simulink model "VSD_Model"  (R2022a)
settings: Solver=VariableStepAuto  StartTime=0.0  StopTime=60
values from neighbouring files (symbols this model uses):
  Bm = 7.33*10^-8/(2*pi)    (= 1.16660573286e-08)    [VSD_Motors_initialization.m]
  fit_Cp_tail = @(u)feval(f_Cp_tail,u)    [VSD_Propellerfitting_tail.m]
  fit_Ct_tail = @(u)feval(f_Ct_tail,u)    [VSD_Propellerfitting_tail.m]
  fit_Pe_tail = @(u)feval(f_Pe_tail,u)    [VSD_Propellerfitting_tail.m]
  fit_Tl_tail = @(u)feval(f_Tl_tail,u)    [VSD_Propellerfitting_tail.m]
  Jm = 1.72 *10^-6    (= 1.72e-06)    [VSD_Motors_initialization.m]
  Ke = Km    (= 0.00118)    [VSD_Motors_initialization.m]
  Km = 1.18*10^-3    (= 0.00118)    [VSD_Motors_initialization.m]
  La = 0.274*10^-3    (= 0.000274)    [VSD_Motors_initialization.m]
  Q = 1e-6    (= 1e-06)    [VSD_initialization.m]
  R = 0.486    [VSD_Motors_initialization.m]    (also in VSD_initialization.m = 0.001)
  Ts = 1e-4    (= 0.0001)    [VSD_initialization.m]    (also in myStateTransitionFcn.m = 0.01)
  x0 = [0;0;0;0;0;0;0;0;0;0;0;0]    [VSD_SystemCheck.m]    (also in VSD_initialization.m = [0,0,0,0,0,0,0,0,0,0,0,0])
undefined symbols (not defined in the file or in its folder): Continuous, Time
libraries: slpidlib x7, simulink x7, sharedTrackingLibrary x3, ctrlSharedLib x1
(part 2 of 2)

== system VSD_Model/Control Allocation Subsystem/DC Motors/Motor21 ==
  w1_ref : Inport
  Tload : Inport  Port=2
  DC Motor : Subsystem
  PID Controller : slpidlib/PID Controller  Controller=PID  Form=Parallel  TimeDomain=Continuous-time  UseExternalTs=off  SampleTime=-1  IntegratorMethod=Forward Euler  FilterMethod=Forward Euler  ControllerParametersSource=internal  P=0.0221631801492144  I=0.197988325342969  UseKiTs=off  D=-5.9672220338915e-06  N=3714.15375920925  UseFilter=on  TunerSelectOption=Transfer Function Based (PID Tuner App)  InitialConditionSource=internal  InitialConditionForIntegrator=0  InitialConditionForFilter=0  DifferentiatorICPrevScaledInput=0  ExternalReset=none  TrackingMode=off  Kt=1  LimitOutput=off  SatLimitsSource=internal  UpperSaturationLimit=inf  LowerSaturationLimit=-inf  LinearizeAsGain=on  AntiWindupMode=none  Kb=1  POutMin=[]  POutMax=[]  IOutMin=[]  IOutMax=[]  DOutMin=[]  DOutMax=[]  NOutMin=[]  NOutMax=[]  SumOutMin=[]  SumOutMax=[]  SaturationOutMin=[]  SaturationOutMax=[]  PParamMin=[]  PParamMax=[]  IParamMin=[]  IParamMax=[]  DParamMin=[]  DParamMax=[]  NParamMin=[]  NParamMax=[]  KbParamMin=[]  KbParamMax=[]  KtParamMin=[]  KtParamMax=[]  KbOutMin=[]  KbOutMax=[]  KtOutMin=[]  KtOutMax=[]  IntegratorOutMin=[]  IntegratorOutMax=[]  FilterOutMin=[]  FilterOutMax=[]  SumI1OutMin=[]  SumI1OutMax=[]  SumI2OutMin=[]  SumI2OutMax=[]  SumI3OutMin=[]  SumI3OutMax=[]  SumI4OutMin=[]  SumI4OutMax=[]  SumDOutMin=[]  SumDOutMax=[]  DifferentiatorOutMin=[]  DifferentiatorOutMax=[]  FilterDiffOutCoefMin=[]  FilterDiffOutCoefMax=[]  ReciprocalOutMin=[]  ReciprocalOutMax=[]  SumDenOutMin=[]  SumDenOutMax=[]  SumNumOutMin=[]  SumNumOutMax=[]  DivideOutMin=[]  DivideOutMax=[]  UdiffTsProdOutMin=[]  UdiffTsProdOutMax=[]  NTsProdOutMin=[]  NTsProdOutMax=[]  UintegralTsProdOutMin=[]  UintegralTsProdOutMax=[]  UngainTsProdOutMin=[]  UngainTsProdOutMax=[]  IntegratorContinuousStateAttributes=''  IntegratorStateMustResolveToSignalObject=off  IntegratorRTWStateStorageClass=Auto  FilterContinuousStateAttributes=''  FilterStateMustResolveToSignalObject=off  FilterRTWStateStorageClass=Auto  ParallelPVariant=InternalParameters  IdealPVariant=Disabled  IVariant=InternalParameters  DVariant=InternalParameters  IntegratorVariant=Continuous  SatVariant=Disabled  AWVariant=Passthrough  PCopyVariant=Disabled  TRVariant=Disabled  FdbkBlocksVariant=Forward  IdealPFdbkVariant=Disabled  SatFdbkVariant=Disabled  DerivativeFilterVariant=ContFilter  NVariant=InternalParameters  NCopyVariant=Disabled  FilterICVariant=InternalICsFilter  IntegratorICVariant=InternalICs  ExternalResetVariant=Disabled  TRSumVariant=Passthrough  SumFdbkVariant=Disabled  SumVariant=Sum_PID  TsampFilterVariant=InternalTs  TsampNgainVariant=Passthrough  TsampIntegralVariant=Passthrough  ExternalSaturationOutDataTypeStr=Inherit: Same as second input  aMode=0
  Step : Step  Time=0  After=0.0015  SampleTime=0
  Sum : Sum  Inputs=|+-
  Theta_dot : Outport
  i1 : Outport  Port=2
  V1 : Outport  Port=3
  wires:
  Sum/1 -> PID Controller/1
  Tload/1 -> DC Motor/2(Tload)
  Step/1 -> DC Motor/3(T_S)
  PID Controller/1 -> DC Motor/1(Vm), V1/1
  DC Motor/2(ia) -> i1/1
  w1_ref/1 -> Sum/1
  DC Motor/1(Theta_dot) -> Theta_dot/1, Sum/2

== system VSD_Model/Control Allocation Subsystem/DC Motors/Motor22 ==
  w3_ref : Inport
  Tload : Inport  Port=2
  DC Motor : Subsystem
  PID Controller : slpidlib/PID Controller  Controller=PID  Form=Parallel  TimeDomain=Continuous-time  UseExternalTs=off  SampleTime=-1  IntegratorMethod=Forward Euler  FilterMethod=Forward Euler  ControllerParametersSource=internal  P=0.0221631801492144  I=0.197988325342969  UseKiTs=off  D=-5.9672220338915e-06  N=3714.15375920925  UseFilter=on  TunerSelectOption=Transfer Function Based (PID Tuner App)  InitialConditionSource=internal  InitialConditionForIntegrator=0  InitialConditionForFilter=0  DifferentiatorICPrevScaledInput=0  ExternalReset=none  TrackingMode=off  Kt=1  LimitOutput=off  SatLimitsSource=internal  UpperSaturationLimit=inf  LowerSaturationLimit=-inf  LinearizeAsGain=on  AntiWindupMode=none  Kb=1  POutMin=[]  POutMax=[]  IOutMin=[]  IOutMax=[]  DOutMin=[]  DOutMax=[]  NOutMin=[]  NOutMax=[]  SumOutMin=[]  SumOutMax=[]  SaturationOutMin=[]  SaturationOutMax=[]  PParamMin=[]  PParamMax=[]  IParamMin=[]  IParamMax=[]  DParamMin=[]  DParamMax=[]  NParamMin=[]  NParamMax=[]  KbParamMin=[]  KbParamMax=[]  KtParamMin=[]  KtParamMax=[]  KbOutMin=[]  KbOutMax=[]  KtOutMin=[]  KtOutMax=[]  IntegratorOutMin=[]  IntegratorOutMax=[]  FilterOutMin=[]  FilterOutMax=[]  SumI1OutMin=[]  SumI1OutMax=[]  SumI2OutMin=[]  SumI2OutMax=[]  SumI3OutMin=[]  SumI3OutMax=[]  SumI4OutMin=[]  SumI4OutMax=[]  SumDOutMin=[]  SumDOutMax=[]  DifferentiatorOutMin=[]  DifferentiatorOutMax=[]  FilterDiffOutCoefMin=[]  FilterDiffOutCoefMax=[]  ReciprocalOutMin=[]  ReciprocalOutMax=[]  SumDenOutMin=[]  SumDenOutMax=[]  SumNumOutMin=[]  SumNumOutMax=[]  DivideOutMin=[]  DivideOutMax=[]  UdiffTsProdOutMin=[]  UdiffTsProdOutMax=[]  NTsProdOutMin=[]  NTsProdOutMax=[]  UintegralTsProdOutMin=[]  UintegralTsProdOutMax=[]  UngainTsProdOutMin=[]  UngainTsProdOutMax=[]  IntegratorContinuousStateAttributes=''  IntegratorStateMustResolveToSignalObject=off  IntegratorRTWStateStorageClass=Auto  FilterContinuousStateAttributes=''  FilterStateMustResolveToSignalObject=off  FilterRTWStateStorageClass=Auto  ParallelPVariant=InternalParameters  IdealPVariant=Disabled  IVariant=InternalParameters  DVariant=InternalParameters  IntegratorVariant=Continuous  SatVariant=Disabled  AWVariant=Passthrough  PCopyVariant=Disabled  TRVariant=Disabled  FdbkBlocksVariant=Forward  IdealPFdbkVariant=Disabled  SatFdbkVariant=Disabled  DerivativeFilterVariant=ContFilter  NVariant=InternalParameters  NCopyVariant=Disabled  FilterICVariant=InternalICsFilter  IntegratorICVariant=InternalICs  ExternalResetVariant=Disabled  TRSumVariant=Passthrough  SumFdbkVariant=Disabled  SumVariant=Sum_PID  TsampFilterVariant=InternalTs  TsampNgainVariant=Passthrough  TsampIntegralVariant=Passthrough  ExternalSaturationOutDataTypeStr=Inherit: Same as second input  aMode=0
  Step : Step  Time=0  After=0.0015  SampleTime=0
  Sum : Sum  Inputs=|+-
  Theta_dot : Outport
  i1 : Outport  Port=2
  V1 : Outport  Port=3
  wires:
  Sum/1 -> PID Controller/1
  Tload/1 -> DC Motor/2(Tload)
  Step/1 -> DC Motor/3(T_S)
  PID Controller/1 -> DC Motor/1(Vm), V1/1
  DC Motor/2(ia) -> i1/1
  w3_ref/1 -> Sum/1
  DC Motor/1(Theta_dot) -> Theta_dot/1, Sum/2

== system VSD_Model/Control Allocation Subsystem/DC Motors/Motor23 ==
  w4_ref : Inport
  Tload : Inport  Port=2
  DC Motor : Subsystem
  PID Controller : slpidlib/PID Controller  Controller=PID  Form=Parallel  TimeDomain=Continuous-time  UseExternalTs=off  SampleTime=-1  IntegratorMethod=Forward Euler  FilterMethod=Forward Euler  ControllerParametersSource=internal  P=0.0221631801492144  I=0.197988325342969  UseKiTs=off  D=-5.9672220338915e-06  N=3714.15375920925  UseFilter=on  TunerSelectOption=Transfer Function Based (PID Tuner App)  InitialConditionSource=internal  InitialConditionForIntegrator=0  InitialConditionForFilter=0  DifferentiatorICPrevScaledInput=0  ExternalReset=none  TrackingMode=off  Kt=1  LimitOutput=off  SatLimitsSource=internal  UpperSaturationLimit=inf  LowerSaturationLimit=-inf  LinearizeAsGain=on  AntiWindupMode=none  Kb=1  POutMin=[]  POutMax=[]  IOutMin=[]  IOutMax=[]  DOutMin=[]  DOutMax=[]  NOutMin=[]  NOutMax=[]  SumOutMin=[]  SumOutMax=[]  SaturationOutMin=[]  SaturationOutMax=[]  PParamMin=[]  PParamMax=[]  IParamMin=[]  IParamMax=[]  DParamMin=[]  DParamMax=[]  NParamMin=[]  NParamMax=[]  KbParamMin=[]  KbParamMax=[]  KtParamMin=[]  KtParamMax=[]  KbOutMin=[]  KbOutMax=[]  KtOutMin=[]  KtOutMax=[]  IntegratorOutMin=[]  IntegratorOutMax=[]  FilterOutMin=[]  FilterOutMax=[]  SumI1OutMin=[]  SumI1OutMax=[]  SumI2OutMin=[]  SumI2OutMax=[]  SumI3OutMin=[]  SumI3OutMax=[]  SumI4OutMin=[]  SumI4OutMax=[]  SumDOutMin=[]  SumDOutMax=[]  DifferentiatorOutMin=[]  DifferentiatorOutMax=[]  FilterDiffOutCoefMin=[]  FilterDiffOutCoefMax=[]  ReciprocalOutMin=[]  ReciprocalOutMax=[]  SumDenOutMin=[]  SumDenOutMax=[]  SumNumOutMin=[]  SumNumOutMax=[]  DivideOutMin=[]  DivideOutMax=[]  UdiffTsProdOutMin=[]  UdiffTsProdOutMax=[]  NTsProdOutMin=[]  NTsProdOutMax=[]  UintegralTsProdOutMin=[]  UintegralTsProdOutMax=[]  UngainTsProdOutMin=[]  UngainTsProdOutMax=[]  IntegratorContinuousStateAttributes=''  IntegratorStateMustResolveToSignalObject=off  IntegratorRTWStateStorageClass=Auto  FilterContinuousStateAttributes=''  FilterStateMustResolveToSignalObject=off  FilterRTWStateStorageClass=Auto  ParallelPVariant=InternalParameters  IdealPVariant=Disabled  IVariant=InternalParameters  DVariant=InternalParameters  IntegratorVariant=Continuous  SatVariant=Disabled  AWVariant=Passthrough  PCopyVariant=Disabled  TRVariant=Disabled  FdbkBlocksVariant=Forward  IdealPFdbkVariant=Disabled  SatFdbkVariant=Disabled  DerivativeFilterVariant=ContFilter  NVariant=InternalParameters  NCopyVariant=Disabled  FilterICVariant=InternalICsFilter  IntegratorICVariant=InternalICs  ExternalResetVariant=Disabled  TRSumVariant=Passthrough  SumFdbkVariant=Disabled  SumVariant=Sum_PID  TsampFilterVariant=InternalTs  TsampNgainVariant=Passthrough  TsampIntegralVariant=Passthrough  ExternalSaturationOutDataTypeStr=Inherit: Same as second input  aMode=0
  Step : Step  Time=0  After=0.0015  SampleTime=0
  Sum : Sum  Inputs=|+-
  Theta_dot : Outport
  i1 : Outport  Port=2
  V1 : Outport  Port=3
  wires:
  Sum/1 -> PID Controller/1
  Tload/1 -> DC Motor/2(Tload)
  Step/1 -> DC Motor/3(T_S)
  PID Controller/1 -> DC Motor/1(Vm), V1/1
  DC Motor/2(ia) -> i1/1
  w4_ref/1 -> Sum/1
  DC Motor/1(Theta_dot) -> Theta_dot/1, Sum/2

== system VSD_Model/Control Allocation Subsystem/DC Motors/Motor24 ==
  w5_ref : Inport
  Tload : Inport  Port=2
  DC Motor : Subsystem
  PID Controller : slpidlib/PID Controller  Controller=PID  Form=Parallel  TimeDomain=Continuous-time  UseExternalTs=off  SampleTime=-1  IntegratorMethod=Forward Euler  FilterMethod=Forward Euler  ControllerParametersSource=internal  P=0.0221631801492144  I=0.197988325342969  UseKiTs=off  D=-5.9672220338915e-06  N=3714.15375920925  UseFilter=on  TunerSelectOption=Transfer Function Based (PID Tuner App)  InitialConditionSource=internal  InitialConditionForIntegrator=0  InitialConditionForFilter=0  DifferentiatorICPrevScaledInput=0  ExternalReset=none  TrackingMode=off  Kt=1  LimitOutput=off  SatLimitsSource=internal  UpperSaturationLimit=inf  LowerSaturationLimit=-inf  LinearizeAsGain=on  AntiWindupMode=none  Kb=1  POutMin=[]  POutMax=[]  IOutMin=[]  IOutMax=[]  DOutMin=[]  DOutMax=[]  NOutMin=[]  NOutMax=[]  SumOutMin=[]  SumOutMax=[]  SaturationOutMin=[]  SaturationOutMax=[]  PParamMin=[]  PParamMax=[]  IParamMin=[]  IParamMax=[]  DParamMin=[]  DParamMax=[]  NParamMin=[]  NParamMax=[]  KbParamMin=[]  KbParamMax=[]  KtParamMin=[]  KtParamMax=[]  KbOutMin=[]  KbOutMax=[]  KtOutMin=[]  KtOutMax=[]  IntegratorOutMin=[]  IntegratorOutMax=[]  FilterOutMin=[]  FilterOutMax=[]  SumI1OutMin=[]  SumI1OutMax=[]  SumI2OutMin=[]  SumI2OutMax=[]  SumI3OutMin=[]  SumI3OutMax=[]  SumI4OutMin=[]  SumI4OutMax=[]  SumDOutMin=[]  SumDOutMax=[]  DifferentiatorOutMin=[]  DifferentiatorOutMax=[]  FilterDiffOutCoefMin=[]  FilterDiffOutCoefMax=[]  ReciprocalOutMin=[]  ReciprocalOutMax=[]  SumDenOutMin=[]  SumDenOutMax=[]  SumNumOutMin=[]  SumNumOutMax=[]  DivideOutMin=[]  DivideOutMax=[]  UdiffTsProdOutMin=[]  UdiffTsProdOutMax=[]  NTsProdOutMin=[]  NTsProdOutMax=[]  UintegralTsProdOutMin=[]  UintegralTsProdOutMax=[]  UngainTsProdOutMin=[]  UngainTsProdOutMax=[]  IntegratorContinuousStateAttributes=''  IntegratorStateMustResolveToSignalObject=off  IntegratorRTWStateStorageClass=Auto  FilterContinuousStateAttributes=''  FilterStateMustResolveToSignalObject=off  FilterRTWStateStorageClass=Auto  ParallelPVariant=InternalParameters  IdealPVariant=Disabled  IVariant=InternalParameters  DVariant=InternalParameters  IntegratorVariant=Continuous  SatVariant=Disabled  AWVariant=Passthrough  PCopyVariant=Disabled  TRVariant=Disabled  FdbkBlocksVariant=Forward  IdealPFdbkVariant=Disabled  SatFdbkVariant=Disabled  DerivativeFilterVariant=ContFilter  NVariant=InternalParameters  NCopyVariant=Disabled  FilterICVariant=InternalICsFilter  IntegratorICVariant=InternalICs  ExternalResetVariant=Disabled  TRSumVariant=Passthrough  SumFdbkVariant=Disabled  SumVariant=Sum_PID  TsampFilterVariant=InternalTs  TsampNgainVariant=Passthrough  TsampIntegralVariant=Passthrough  ExternalSaturationOutDataTypeStr=Inherit: Same as second input  aMode=0
  Step : Step  Time=0  After=0.0015  SampleTime=0
  Sum : Sum  Inputs=|+-
  Theta_dot : Outport
  i1 : Outport  Port=2
  V1 : Outport  Port=3
  wires:
  Sum/1 -> PID Controller/1
  Tload/1 -> DC Motor/2(Tload)
  Step/1 -> DC Motor/3(T_S)
  PID Controller/1 -> DC Motor/1(Vm), V1/1
  DC Motor/2(ia) -> i1/1
  w5_ref/1 -> Sum/1
  DC Motor/1(Theta_dot) -> Theta_dot/1, Sum/2

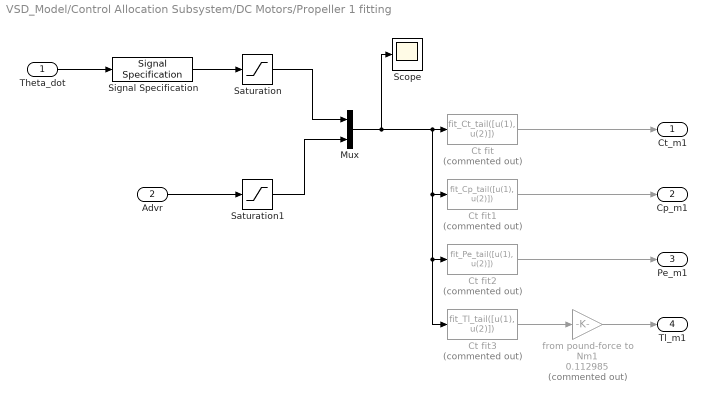
== system VSD_Model/Control Allocation Subsystem/DC Motors/Propeller 1 fitting ==
  Theta_dot : Inport
  Advr : Inport  Port=2
  Ct fit : MATLABFcn  Commented=on  MATLABFcn=fit_Ct_tail([u(1), u(2)])
  Ct fit1 : MATLABFcn  Commented=on  MATLABFcn=fit_Cp_tail([u(1), u(2)])
  Ct fit2 : MATLABFcn  Commented=on  MATLABFcn=fit_Pe_tail([u(1), u(2)])
  Ct fit3 : MATLABFcn  Commented=on  MATLABFcn=fit_Tl_tail([u(1), u(2)])
  Mux : Mux  Inputs=2
  Saturation : Saturate  UpperLimit=15000  LowerLimit=1000
  Saturation1 : Saturate  UpperLimit=1.07  LowerLimit=0
  Scope : Scope
  Signal Specification : SignalSpecification  Dimensions=1
  from pound-force to Nm1 : Gain  Commented=on  Gain=0.112985
  Ct_m1 : Outport
  Cp_m1 : Outport  Port=2
  Pe_m1 : Outport  Port=3
  Tl_m1 : Outport  Port=4
  wires:
  Advr/1 -> Saturation1/1
  Saturation/1 -> Mux/1
  Saturation1/1 -> Mux/2
  Mux/1 -> Scope/1, Ct fit/1, Ct fit1/1, Ct fit3/1, Ct fit2/1
  Ct fit/1 -> Ct_m1/1
  Ct fit2/1 -> Pe_m1/1
  Ct fit1/1 -> Cp_m1/1
  Signal Specification/1 -> Saturation/1
  Theta_dot/1 -> Signal Specification/1
  Ct fit3/1 -> from pound-force to Nm1/1
  from pound-force to Nm1/1 -> Tl_m1/1

== system VSD_Model/UAV Dynamics/Drag and Wind Disturbances/Drag Forces ==
  u : Inport
  Input : Inport  Port=2
  Gain : Gain  Gain=1/1.331
  MATLAB Function : MATLAB Function  TreatAsAtomicUnit=on
  Fdi : Outport
  wires:
  u/1 -> MATLAB Function/1(vi)  "vi"
  Input/1 -> MATLAB Function/2(ai)
  Gain/1 -> Fdi/1
  MATLAB Function/1(Fdi) -> Gain/1

== system VSD_Model/UAV Dynamics/Drag and Wind Disturbances/Wind Forces ==
  Input : Inport
  Input1 : Inport  Port=2
  Gain : Gain  Gain=1.331
  MATLAB Function : MATLAB Function  TreatAsAtomicUnit=on
  Fdi : Outport
  wires:
  Gain/1 -> Fdi/1
  MATLAB Function/1(Fwi) -> Gain/1
  Input/1 -> MATLAB Function/2(ai)
  Input1/1 -> MATLAB Function/1(vw)

== system VSD_Model/Control Allocation Subsystem/DC Motors/Motor/DC Motor ==
  Vm : Inport
  Tload : Inport  Port=2
  T_S : Inport  Port=3
  Armature1 : TransferFcn  Denominator=[La R]
  Gain1 : Gain  Gain=Ke
  Motor1 : TransferFcn  Denominator=[Jm Bm]
  Sum1 : Sum  Inputs=-+|
  Sum7 : Sum  Inputs=-+|
  Sum9 : Sum  Inputs=|+-
  km : Gain  Gain=Km
  Theta_dot : Outport
  ia : Outport  Port=2
  wires:
  Sum9/1 -> Armature1/1
  Gain1/1 -> Sum9/2
  Armature1/1 -> ia/1, km/1  "ia"
  Motor1/1 -> Theta_dot/1, Gain1/1  "theta_dot"
  Tload/1 -> Sum7/1
  Sum7/1 -> Motor1/1
  Sum1/1 -> Sum7/2
  km/1 -> Sum1/2  "Tm"
  T_S/1 -> Sum1/1
  Vm/1 -> Sum9/1

== system VSD_Model/Control Allocation Subsystem/DC Motors/Motor1/DC Motor ==
  Vm : Inport
  Tload : Inport  Port=2
  T_S : Inport  Port=3
  Armature1 : TransferFcn  Denominator=[La R]
  Gain1 : Gain  Gain=Ke
  Integrator : Integrator
  Motor1 : TransferFcn  Denominator=[Jm Bm]
  Sum1 : Sum  Inputs=-+|
  Sum7 : Sum  Inputs=-+|
  Sum9 : Sum  Inputs=|+-
  km : Gain  Gain=Km
  alpha_l : Outport
  ia : Outport  Port=2
  wires:
  Sum9/1 -> Armature1/1
  Gain1/1 -> Sum9/2
  Armature1/1 -> ia/1, km/1  "ia"
  Motor1/1 -> Integrator/1, Gain1/1  "theta_dot"
  Tload/1 -> Sum7/1
  Sum7/1 -> Motor1/1
  Sum1/1 -> Sum7/2
  km/1 -> Sum1/2  "Tm"
  T_S/1 -> Sum1/1
  Vm/1 -> Sum9/1
  Integrator/1 -> alpha_l/1

== system VSD_Model/Control Allocation Subsystem/DC Motors/Motor2/DC Motor ==
  Vm : Inport
  Tload : Inport  Port=2
  T_S : Inport  Port=3
  Armature1 : TransferFcn  Denominator=[La R]
  Gain1 : Gain  Gain=Ke
  Integrator : Integrator
  Motor1 : TransferFcn  Denominator=[Jm Bm]
  Sum1 : Sum  Inputs=-+|
  Sum7 : Sum  Inputs=-+|
  Sum9 : Sum  Inputs=|+-
  km : Gain  Gain=Km
  Theta : Outport
  ia : Outport  Port=2
  wires:
  Sum9/1 -> Armature1/1
  Gain1/1 -> Sum9/2
  Armature1/1 -> ia/1, km/1  "ia"
  Motor1/1 -> Gain1/1, Integrator/1  "theta_dot"
  Tload/1 -> Sum7/1
  Sum7/1 -> Motor1/1
  Sum1/1 -> Sum7/2
  km/1 -> Sum1/2  "Tm"
  T_S/1 -> Sum1/1
  Vm/1 -> Sum9/1
  Integrator/1 -> Theta/1

== system VSD_Model/Control Allocation Subsystem/DC Motors/Motor21/DC Motor ==
  Vm : Inport
  Tload : Inport  Port=2
  T_S : Inport  Port=3
  Armature1 : TransferFcn  Denominator=[La R]
  Gain1 : Gain  Gain=Ke
  Motor1 : TransferFcn  Denominator=[Jm Bm]
  Sum1 : Sum  Inputs=-+|
  Sum7 : Sum  Inputs=-+|
  Sum9 : Sum  Inputs=|+-
  km : Gain  Gain=Km
  Theta_dot : Outport
  ia : Outport  Port=2
  wires:
  Sum9/1 -> Armature1/1
  Gain1/1 -> Sum9/2
  Armature1/1 -> ia/1, km/1  "ia"
  Motor1/1 -> Theta_dot/1, Gain1/1  "theta_dot"
  Tload/1 -> Sum7/1
  Sum7/1 -> Motor1/1
  Sum1/1 -> Sum7/2
  km/1 -> Sum1/2  "Tm"
  T_S/1 -> Sum1/1
  Vm/1 -> Sum9/1

== system VSD_Model/Control Allocation Subsystem/DC Motors/Motor22/DC Motor ==
  Vm : Inport
  Tload : Inport  Port=2
  T_S : Inport  Port=3
  Armature1 : TransferFcn  Denominator=[La R]
  Gain1 : Gain  Gain=Ke
  Motor1 : TransferFcn  Denominator=[Jm Bm]
  Sum1 : Sum  Inputs=-+|
  Sum7 : Sum  Inputs=-+|
  Sum9 : Sum  Inputs=|+-
  km : Gain  Gain=Km
  Theta_dot : Outport
  ia : Outport  Port=2
  wires:
  Sum9/1 -> Armature1/1
  Gain1/1 -> Sum9/2
  Armature1/1 -> ia/1, km/1  "ia"
  Motor1/1 -> Theta_dot/1, Gain1/1  "theta_dot"
  Tload/1 -> Sum7/1
  Sum7/1 -> Motor1/1
  Sum1/1 -> Sum7/2
  km/1 -> Sum1/2  "Tm"
  T_S/1 -> Sum1/1
  Vm/1 -> Sum9/1

== system VSD_Model/Control Allocation Subsystem/DC Motors/Motor23/DC Motor ==
  Vm : Inport
  Tload : Inport  Port=2
  T_S : Inport  Port=3
  Armature1 : TransferFcn  Denominator=[La R]
  Gain1 : Gain  Gain=Ke
  Motor1 : TransferFcn  Denominator=[Jm Bm]
  Sum1 : Sum  Inputs=-+|
  Sum7 : Sum  Inputs=-+|
  Sum9 : Sum  Inputs=|+-
  km : Gain  Gain=Km
  Theta_dot : Outport
  ia : Outport  Port=2
  wires:
  Sum9/1 -> Armature1/1
  Gain1/1 -> Sum9/2
  Armature1/1 -> ia/1, km/1  "ia"
  Motor1/1 -> Theta_dot/1, Gain1/1  "theta_dot"
  Tload/1 -> Sum7/1
  Sum7/1 -> Motor1/1
  Sum1/1 -> Sum7/2
  km/1 -> Sum1/2  "Tm"
  T_S/1 -> Sum1/1
  Vm/1 -> Sum9/1

== system VSD_Model/Control Allocation Subsystem/DC Motors/Motor24/DC Motor ==
  Vm : Inport
  Tload : Inport  Port=2
  T_S : Inport  Port=3
  Armature1 : TransferFcn  Denominator=[La R]
  Gain1 : Gain  Gain=Ke
  Motor1 : TransferFcn  Denominator=[Jm Bm]
  Sum1 : Sum  Inputs=-+|
  Sum7 : Sum  Inputs=-+|
  Sum9 : Sum  Inputs=|+-
  km : Gain  Gain=Km
  Theta_dot : Outport
  ia : Outport  Port=2
  wires:
  Sum9/1 -> Armature1/1
  Gain1/1 -> Sum9/2
  Armature1/1 -> ia/1, km/1  "ia"
  Motor1/1 -> Theta_dot/1, Gain1/1  "theta_dot"
  Tload/1 -> Sum7/1
  Sum7/1 -> Motor1/1
  Sum1/1 -> Sum7/2
  km/1 -> Sum1/2  "Tm"
  T_S/1 -> Sum1/1
  Vm/1 -> Sum9/1

== matlab function VSD_Model/Control Allocation Subsystem/Control allocation/MATLAB Function1 ==
  data: u input; y output
function y = fcn(u)

y = u^(1/4);

== matlab function VSD_Model/Reference Generator/Position References (HELIX // RAMP) ==
  data: t input; x_des output; dx_des output; ddx_des output; y_des output; dy_des output; ddy_des output; z_des output; dz_des output; ddz_des output
function [x_des, dx_des, ddx_des, y_des, dy_des, ddy_des, z_des, dz_des, ddz_des]  = fcn(t)

% % Trajectory: HELIX
x_des = sin(t);
y_des = cos(t);
z_des = t;

dx_des = cos(t);
dy_des = -sin(t);
dz_des = 1;

ddx_des = -sin(t);
ddy_des = -cos(t);
ddz_des = 0;

% % Trajectory: RAMP + CONSTANT MOTION X-AXIS
% x_des = t;
% y_des = 1;
% z_des = 5;
% 
% dx_des = 1;
% dy_des = 0;
% dz_des = 0;
% 
% ddx_des = 0;
% ddy_des = 0;
% ddz_des = 0;

% % Trajectory: HOVERING
% x_des = 0;
% y_des = 0;
% z_des = t;
% 
% dx_des = 0;
% dy_des = 0;
% dz_des = 1;
% 
% ddx_des = 0;
% ddy_des = 0;
% ddz_des = 0;

% % Trajectory: SINUSOID ON Z-AXIS
% x_des = t;
% y_des = 0;
% z_des = 5 + sin(t);
% 
% dx_des = 1;
% dy_des = 0;
% dz_des = cos(t);
% 
% ddx_des = 0;
% ddy_des = 0;
% ddz_des = 0;

== matlab function VSD_Model/Control Allocation Subsystem/Control allocation/MATLAB Function2 ==
  data: u input; y output
function y = fcn(u)

y = u^(1/4);

== matlab function VSD_Model/UAV Dynamics/Drag and Wind Disturbances/Drag Forces/MATLAB Function ==
  data: vi input; Fdi output size=3; ai input
function Fdi = fcn(vi, ai)
rho = 1.18;
Ax = 8.59e-3;
Ay = 15.48e-3;
Az = 29.11e-3;
Cdx = 0.06277;
Cdy = 0.03221;
Cdz = 0.04952;

vx = vi(1);
vy = vi(2);
vz = vi(3);

phi = ai(1);
tht = ai(2);
psi = ai(3);

Rotbi=[cos(tht)*cos(psi) sin(tht)*cos(psi)*sin(phi)-sin(psi)*cos(phi) sin(tht)*cos(psi)*cos(phi)+sin(psi)*sin(phi);
              cos(tht)*sin(psi) sin(tht)*sin(psi)*sin(phi)+cos(psi)*cos(phi) sin(tht)*sin(psi)*cos(phi)-cos(psi)*sin(phi);
              -sin(tht)            cos(tht)*sin(phi)                                     cos(tht)*cos(phi);];

          
 vb = inv(Rotbi)*[vx; vy; vz];
 
vbx=vb(1); vby=vb(2); vbz=vb(3);

 
Fdx = 0.5*rho*Ax*Cdx*(vbx^2);
Fdy = 0.5*rho*Ay*Cdy*(vby^2);
Fdz = 0.5*rho*Az*Cdz*(vbz^2);

Fdb = [Fdx; Fdy; Fdz];

Fdi = Rotbi*Fdb;

== matlab function VSD_Model/UAV Dynamics/Drag and Wind Disturbances/Wind Forces/MATLAB Function ==
  data: vw input; Fwi output; ai input
function Fwi = fcn(vw, ai)
rho = 1.18;
Ax = 8.59e-3;
Ay = 15.48e-3;
Az = 29.11e-3;
Cdx = 0.06277;
Cdy = 0.03221;
Cdz = 0.04952;

vwx = vw(1);
vwy = vw(2);
vwz = vw(3);
phi = ai(1);
tht = ai(2);
psi = ai(3);

Rotbi=[cos(tht)*cos(psi) sin(tht)*cos(psi)*sin(phi)-sin(psi)*cos(phi) sin(tht)*cos(psi)*cos(phi)+sin(psi)*sin(phi);
              cos(tht)*sin(psi) sin(tht)*sin(psi)*sin(phi)+cos(psi)*cos(phi) sin(tht)*sin(psi)*cos(phi)-cos(psi)*sin(phi);
              -sin(tht)            cos(tht)*sin(phi)                                     cos(tht)*cos(phi);];

          
vwb = inv(Rotbi)*[vwx; vwy; vwz];
 
vwbx=vwb(1); vwby=vwb(2); vwbz=vwb(3);


Fwx = 0.5*rho*Ax*Cdx*(vwbx^2);
Fwy = 0.5*rho*Ay*Cdy*(vwby^2);
Fwz = 0.5*rho*Az*Cdz*(vwbz^2);

Fwb = [Fwx; Fwy; Fwz];

Fwi = Rotbi*Fwb;

== matlab function VSD_Model/Postion Controller/Virtual  Controller ==
  data: xref input size=9; u1d output; u2d output; u3d output; x_pos input size=6
function [u1d,u2d,u3d] = fcn(xref,x_pos)
% define the first six inputs as the ref, states from 1 to 6 
x1r=xref(1);
x2r=xref(2);
dx2r=xref(3);
x3r=xref(4);
x4r=xref(5);
dx4r=xref(6);
x5r=xref(7);
x6r=xref(8);
dx6r=xref(9);
% define the second six inputs as the Current , states from 1 to 6 
x1=x_pos(1);
x2=x_pos(2);
x3=x_pos(3);
x4=x_pos(4);
x5=x_pos(5);
x6=x_pos(6);
% define the error 
e1=x1r-x1;
e2=x2r-x2;
e3=x3r-x3;
e4=x4r-x4;
e5=x5r-x5;
e6=x6r-x6;
% define K 
k1=1*3;
k2=2*3;
k3=2*3;
k4=3*3;
k5=1*3;
k6=3*2;
% define the virtual controls 
u1d = e1 + k2*e2 + dx2r;
u2d = e3 + k4*e4 + dx4r;
u3d = e5 + k6*e6 + dx6r;

== matlab function VSD_Model/Attuide Controller/Attitude Controller ==
  data: x_rot input size=6; u4 output; x7r input; dx7r input; x9r input; dx9r input; x11r input; dx11r input; u5 output; u6 output; s output
function [u4,u5,u6,s] = fcn(x_rot,x7r,dx7r,x9r,dx9r,x11r,dx11r)

% k7 = 2;
k7 = 2*5;
k8 = 5*5;
k9 = 3*2;
k10 = 7*2;
k11 = 5;
k12 = 3;

Ixx = 1.03e-2;
Iyy = 9.02e-3;
Izz = 1.72e-2;

a1 = 1/Ixx;
a2 = 1/Iyy;
a3 = 1/Izz;

b1=(Iyy-Izz)/Ixx;
b2=(Izz-Ixx)/Iyy;
b3=(Ixx-Iyy)/Izz;

%ADAPTIVE
eta1=1;
eta2=1;
eta3=1;


x7 = x_rot(1);
x8 = x_rot(2);
x9 = x_rot(3);
x10 = x_rot(4);
x11 = x_rot(5);
x12 = x_rot(6);


% Control u4
e7 = x7r - x7;
x8r = k7*e7 + dx7r;
e8 = k7*e7 + dx7r - x8;
s1 = e8;

dx8r = (1+k7)*dx7r - k7*x8;

u4 = (1/a1)*(e7 + dx8r -b1*x10*x12 + eta1*atan(s1)*(2/pi) + k8*s1);


% Control u5
e9 = x9r - x9;
x10r = k9*e9 + dx9r;
e10 = k9*e9 + dx9r - x10;
s2 = e10;
dx10r = (1+k9)*dx9r - k9*x10;


u5 = (1/a2)*(e9 + dx10r -b2*x8*x12 + eta2*atan(s2)*(2/pi) + k10*s2);

% Control u6
e11 = x11r - x11;
x12r = k11*e11 + dx11r;
e12 = k11*e11 + dx11r - x12;
s3 = e12;
dx12r = (1+k11)*dx11r - k11*x12;


u6 = (1/a3)*(e11 + dx12r -b3*x8*x10 + eta3*atan(s3)*(2/pi) + k12*s3);

s=[s1;s2;s3];

== matlab function VSD_Model/Control Allocation Subsystem/DC Motors/Real Applied inputs ==
  data: u_real input; u_applied output
function u_applied = fcn(u_real)
ctf = 1.63e-5;
ctr = 9.6e-6;
cq = 2.4e-7;

l1 = 0.240;
l2 = 0.078;
l3 = 0.151;

w1 = u_real(1);
w2 = u_real(2);
w3 = u_real(3);
w4 = u_real(4);
w5 = u_real(5);
alpha_l = u_real(6);
alpha_r = u_real(7);



M = [0       0          2*ctf     0          2*ctf;
     -ctr    -2*ctf     0         -2*ctf     0;
     0       -2*ctf*l3  0         2*ctf*l3   0;
     -ctr*l1 2*ctf*l2 0           2*ctf*l3   0;
     0       0        -2*ctf*l3   0          2*ctf*l3;];


u_real1 = w1^2;
u_real2 = w2^2*cos(alpha_r);
u_real3 = w3^2*sin(alpha_r);
u_real4 = w4^2*cos(alpha_l);
u_real5 = w5^2*cos(alpha_l);

u_real_new = [u_real1; u_real2; u_real3; u_real4; u_real5];

u_applied = M*u_real_new;

== matlab function VSD_Model/Sensors Model3/Body 2 Inertial ==
  data: u input; y output; x_if input
function y = fcn(u, x_if)
% Angles in the inertial frame 
phi = x_if(7);
tht = x_if(9);
psi = x_if(11);

% Rotation matrix from body to inertial frames
Rotbi=[cos(tht)*cos(psi) sin(tht)*cos(psi)*sin(phi)-sin(psi)*cos(phi) sin(tht)*cos(psi)*cos(phi)+sin(psi)*sin(phi);
              cos(tht)*sin(psi) sin(tht)*sin(psi)*sin(phi)+cos(psi)*cos(phi) sin(tht)*sin(psi)*cos(phi)-cos(psi)*sin(phi);
              -sin(tht)            cos(tht)*sin(phi)                                     cos(tht)*cos(phi);];

y = Rotbi*u;

== matlab function VSD_Model/Sensors Model1/From Inertial to Body Coordinates ==
  data: v output; x_if input; omega_bf output
function [v, omega_bf] = fcn(x_if)

% Angles in the inertial frame 
phi = x_if(7);
tht = x_if(9);
psi = x_if(11);

% Angular speeds in the inertial frame
phi_dot = x_if(8);
tht_dot = x_if(10);
psi_dot = x_if(12);

% Translational speeds
v = [x_if(2); x_if(4); x_if(6)];

% Rotation matrix from body to inertial frames
Rotbi=[cos(tht)*cos(psi) sin(tht)*cos(psi)*sin(phi)-sin(psi)*cos(phi) sin(tht)*cos(psi)*cos(phi)+sin(psi)*sin(phi);
              cos(tht)*sin(psi) sin(tht)*sin(psi)*sin(phi)+cos(psi)*cos(phi) sin(tht)*sin(psi)*cos(phi)-cos(psi)*sin(phi);
              -sin(tht)            cos(tht)*sin(phi)                                     cos(tht)*cos(phi);];

% Rotation matrix from inertial to body frame
Rotib = inv(Rotbi);

% Angular velocities in the body frame
omega_bf = Rotib*[phi_dot; tht_dot; psi_dot];

% ADD POSITIONS ALSO ????

== matlab function VSD_Model/Sensors Model3/From Body to Inertial Coordinates ==
  data: u input; y output; x_if input
function y = fcn(u, x_if)
% Angles in the inertial frame 
phi = x_if(7);
tht = x_if(9);
psi = x_if(11);

% Rotation matrix from body to inertial frames
Rotbi=[cos(tht)*cos(psi) sin(tht)*cos(psi)*sin(phi)-sin(psi)*cos(phi) sin(tht)*cos(psi)*cos(phi)+sin(psi)*sin(phi);
              cos(tht)*sin(psi) sin(tht)*sin(psi)*sin(phi)+cos(psi)*cos(phi) sin(tht)*sin(psi)*cos(phi)-cos(psi)*sin(phi);
              -sin(tht)            cos(tht)*sin(phi)                                     cos(tht)*cos(phi);];

y = Rotbi*u;

== matlab function VSD_Model/Sensors Model3/From Inertial to Body Coordinates ==
  data: v_bf output; x_if input; omega_bf output
function [v_bf, omega_bf] = fcn(x_if)

% Angles in the inertial frame 
phi = x_if(7);
tht = x_if(9);
psi = x_if(11);

% Angular speeds in the inertial frame
phi_dot = x_if(8);
tht_dot = x_if(10);
psi_dot = x_if(12);

% Translational speeds
v = [x_if(2); x_if(4); x_if(6)];

% Rotation matrix from body to inertial frames
Rotbi=[cos(tht)*cos(psi) sin(tht)*cos(psi)*sin(phi)-sin(psi)*cos(phi) sin(tht)*cos(psi)*cos(phi)+sin(psi)*sin(phi);
              cos(tht)*sin(psi) sin(tht)*sin(psi)*sin(phi)+cos(psi)*cos(phi) sin(tht)*sin(psi)*cos(phi)-cos(psi)*sin(phi);
              -sin(tht)            cos(tht)*sin(phi)                                     cos(tht)*cos(phi);];

% Rotation matrix from inertial to body frame
Rotib = inv(Rotbi);

% Angular velocities in the body frame
omega_bf = Rotib*[phi_dot; tht_dot; psi_dot];
v_bf = Rotib*v;

% ADD POSITIONS ALSO ????

== matlab function VSD_Model/Subsystem/Sensors Model2/Body 2 Inertial ==
  data: u input; y output; x_if input
function y = fcn(u, x_if)
% Angles in the inertial frame 
phi = x_if(7);
tht = x_if(9);
psi = x_if(11);

% Rotation matrix from body to inertial frames
Rotbi=[cos(tht)*cos(psi) sin(tht)*cos(psi)*sin(phi)-sin(psi)*cos(phi) sin(tht)*cos(psi)*cos(phi)+sin(psi)*sin(phi);
              cos(tht)*sin(psi) sin(tht)*sin(psi)*sin(phi)+cos(psi)*cos(phi) sin(tht)*sin(psi)*cos(phi)-cos(psi)*sin(phi);
              -sin(tht)            cos(tht)*sin(phi)                                     cos(tht)*cos(phi);];

y = Rotbi*u;

== matlab function VSD_Model/Subsystem/Sensors Model2/From Body to Inertial Coordinates ==
  data: u input; y output; x_if input
function y = fcn(u, x_if)
% Angles in the inertial frame 
phi = x_if(7);
tht = x_if(9);
psi = x_if(11);

% Rotation matrix from body to inertial frames
Rotbi=[cos(tht)*cos(psi) sin(tht)*cos(psi)*sin(phi)-sin(psi)*cos(phi) sin(tht)*cos(psi)*cos(phi)+sin(psi)*sin(phi);
              cos(tht)*sin(psi) sin(tht)*sin(psi)*sin(phi)+cos(psi)*cos(phi) sin(tht)*sin(psi)*cos(phi)-cos(psi)*sin(phi);
              -sin(tht)            cos(tht)*sin(phi)                                     cos(tht)*cos(phi);];

y = Rotbi*u;

== matlab function VSD_Model/Subsystem/Sensors Model2/From Inertial to Body Coordinates ==
  data: v_bf output; x_if input; omega_bf output
function [v_bf, omega_bf] = fcn(x_if)

% Angles in the inertial frame 
phi = x_if(7);
tht = x_if(9);
psi = x_if(11);

% Angular speeds in the inertial frame
phi_dot = x_if(8);
tht_dot = x_if(10);
psi_dot = x_if(12);

% Translational speeds
v = [x_if(2); x_if(4); x_if(6)];

% Rotation matrix from body to inertial frames
Rotbi=[cos(tht)*cos(psi) sin(tht)*cos(psi)*sin(phi)-sin(psi)*cos(phi) sin(tht)*cos(psi)*cos(phi)+sin(psi)*sin(phi);
              cos(tht)*sin(psi) sin(tht)*sin(psi)*sin(phi)+cos(psi)*cos(phi) sin(tht)*sin(psi)*cos(phi)-cos(psi)*sin(phi);
              -sin(tht)            cos(tht)*sin(phi)                                     cos(tht)*cos(phi);];

% Rotation matrix from inertial to body frame
Rotib = inv(Rotbi);

% Angular velocities in the body frame
omega_bf = Rotib*[phi_dot; tht_dot; psi_dot];

% Linear velocities in the body frame
v_bf = Rotib*v;

== matlab function VSD_Model/UAV Dynamics/Rotation Dynamics ==
  data: x1 input; dx7 output; x2 input; x3 input; x4 input; x5 input; x6 input; x7 input; x8 input; x9 input; x10 input; x11 input; x12 input; u3 input; u4 input; u5 input; dx8 output; dx9 output; dx10 output; dx11 output; dx12 output
function [dx7,dx8,dx9,dx10,dx11,dx12] = fcn(x1,x2,x3,x4,x5,x6,x7,x8,x9,x10,x11,x12,u3,u4,u5)
Ixx = 1.03e-2;
Iyy = 9.02e-3;
Izz = 1.72e-2;

dx7 = x8;
dx8 = (1/Ixx)*(Iyy - Izz)*x10*x12 + (1/Ixx)*u3;
dx9 = x10;
dx10 = (1/Iyy)*(Izz - Ixx)*x8*x12 + (1/Iyy)*u4;
dx11 = x12;
dx12 = (1/Izz)*(Ixx - Iyy)*x8*x10 + (1/Izz)*u5;

== matlab function VSD_Model/UAV Dynamics/Position Dynamics ==
  data: x1 input; dx1 output; x2 input; x3 input; x4 input; x5 input; x6 input; x7 input; x8 input; x9 input; x10 input; x11 input; x12 input; u1 input; u2 input; dx2 output; dx3 output; dx4 output; dx5 output; dx6 output
function [dx1,dx2,dx3,dx4,dx5,dx6] = fcn(x1,x2,x3,x4,x5,x6,x7,x8,x9,x10,x11,x12,u1,u2)
m = 1.331;
g = 9.807;
    
dx1 = x2;
dx2 = (1/m)*cos(x9)*cos(x11)*u1 + (1/m)*(sin(x9)*cos(x11)*cos(x7) + sin(x11)*sin(x7))*u2;
dx3 = x4;
dx4 = (1/m)*cos(x9)*sin(x11)*u1 + (1/m)*(sin(x9)*sin(x11)*cos(x7) - cos(x11)*sin(x7))*u2;
dx5 = x6;
dx6 = g - (1/m)*sin(x9)*u1 + (1/m)*cos(x9)*cos(x7)*u2;

== matlab function VSD_Model/Control Allocation Subsystem/Control allocation/MATLAB Function ==
  data: u input; y output
function y = fcn(u)

ctf = 1.63e-5;
ctr = 9.6e-6;

cq = 2.4e-7;

l1 = 0.240;
l2 = 0.078;
l3 = 0.151;

M = [0       0          2*ctf     0          2*ctf;
     -ctr    -2*ctf     0         -2*ctf     0;
     0       -2*ctf*l3  0         2*ctf*l3   0;
     -ctr*l1 2*ctf*l2 0           2*ctf*l3   0;
     0       0        -2*ctf*l3   0          2*ctf*l3;];
 
M_inv = inv(M);

y = M_inv*u;


% Fbx = u(1);
% Fby = u(2);
% tau_bx = u(3);
% tau_by = u(4);
% tau_bz = u(5);

== matlab function VSD_Model/Postion Controller/Decoupler ==
  data: ud input; x7r output; x7 input; x9 input; x11 input; ux output; uz output
function [x7r,ux,uz] = fcn(ud,x7,x9,x11)
g = 9.807;

ud1=ud(1);
ud2=ud(2);
ud3=ud(3);


x7r = (ud1*sin(x11)-ud2*cos(x11))/(ud1*sin(x9)*cos(x11)+ud2*sin(x9)*sin(x11)+(ud3-g)*cos(x9));
ux = (ud1*cos(x11)+ud2*sin(x11))-(ud3-g)*(sin(x9));
uz = (ud1*sin(x11)-ud2*cos(x11))*sin(x7r)+(ud1*sin(x9)*cos(x11)+ud2*sin(x9)*sin(x11)+(ud3-g)*cos(x9))*cos(x7r);
